simulink subsystem "Find_Control_Pose"  (R2023b)
settings: Solver=VariableStepAuto  StartTime=0.0  StopTime=10.0  RelTol=1e-3
settings Model: Creator=FIRSTMentor  LastModifiedBy=FIRSTMentor

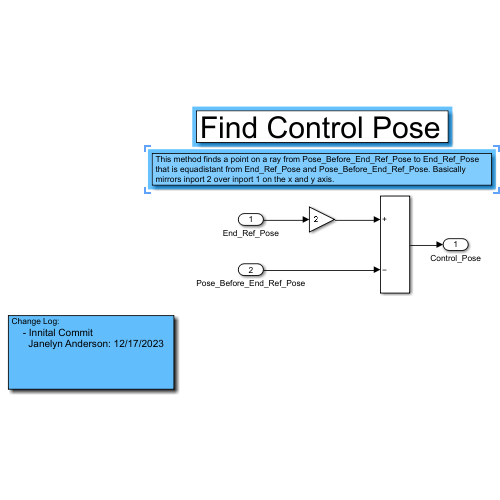
[thumbnail: Simulink's stored preview of the top-level diagram]
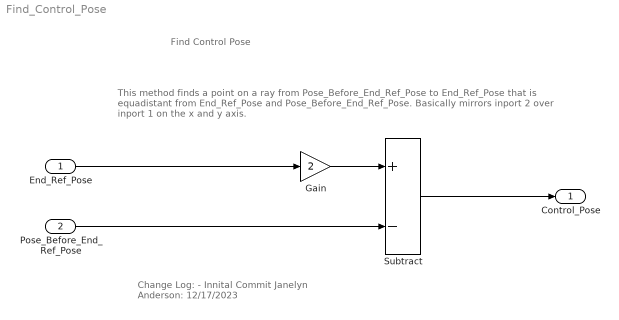
== system Find_Control_Pose ==
  note: Find Control Pose
  note: This method finds a point on a ray from Pose_Before_End_Ref_Pose to End_Ref_Pose that is equadistant from End_Ref_Pose and Pose_Before_End_Ref_Pose. Basically mirrors inport 2 over inport 1 on the x and y axis.
  note: Change Log:
      | - Innital Commit
      | Janelyn Anderson: 12/17/2023
  End_Ref_Pose : Inport
  Pose_Before_End_Ref_Pose : Inport  Port=2
  Gain : Gain  Gain=2
  Subtract : Sum  Inputs=+-
  Control_Pose : Outport
  wires:
  Subtract/1 -> Control_Pose/1
  Gain/1 -> Subtract/1
  End_Ref_Pose/1 -> Gain/1
  Pose_Before_End_Ref_Pose/1 -> Subtract/2
